simulink model "SISTEMA5_3"  (R2025b)
settings: Solver=VariableStepAuto  StartTime=0.0  StopTime=10.0  RelTol=1e-3
libraries: slpidlib x2

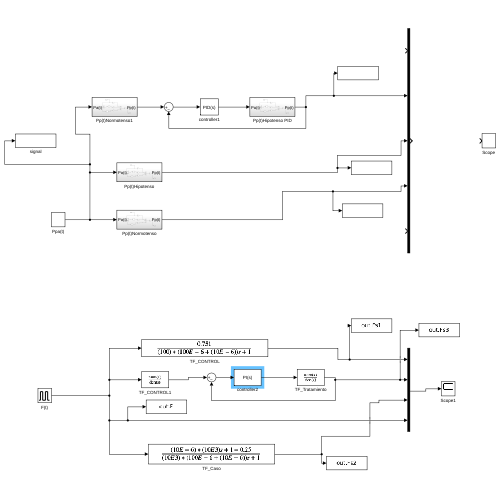
[thumbnail: Simulink's stored preview of the top-level diagram]
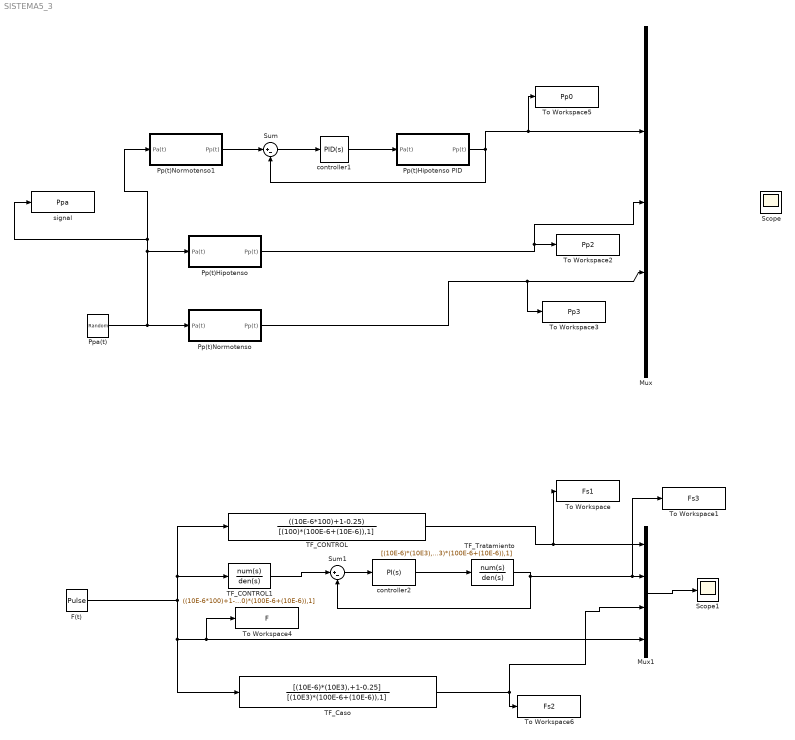
== system SISTEMA5_3 ==
  F(t) : DiscretePulseGenerator  PulseType=Time based  Period=10  PulseWidth=10  PhaseDelay=1
  Mux : Mux  Inputs=5
  Mux1 : Mux
  Pp(t)Hipotenso : Subsystem
  Pp(t)Hipotenso PID : Subsystem
  Pp(t)Normotenso : Subsystem
  Pp(t)Normotenso1 : Subsystem
  Ppa(t) : UniformRandomNumber  Minimum=-0.2  Seed=106  SampleTime=0.5
  Scope : Scope
  Scope1 : Scope
      settings: ActiveDisplayYMinimum=-0.12525889931530931  ActiveDisplayYMaximum=1.2530462249099128
  Sum : Sum  Inputs=|+-
  Sum1 : Sum  Inputs=|+-
  TF_CONTROL : TransferFcn  Numerator=((10E-6*100)+1-0.25)  Denominator=[(100)*(100E-6+(10E-6)),1]
  TF_CONTROL1 : TransferFcn  Numerator=((10E-6*100)+1-0.25)  Denominator=[(100)*(100E-6+(10E-6)),1]
  TF_Caso : TransferFcn  Numerator=[(10E-6)*(10E3),+1-0.25]  Denominator=[(10E3)*(100E-6+(10E-6)),1]
  TF_Tratamiento : TransferFcn  Numerator=[(10E-6)*(10E3),+1-0.25]  Denominator=[(10E3)*(100E-6+(10E-6)),1]
  To Workspace : ToWorkspace  VariableName=Fs1  SampleTime=-1
      settings: Save2DSignal=2-D array (concatenate along first dimension)
  To Workspace1 : ToWorkspace  VariableName=Fs3  SampleTime=-1
      settings: Save2DSignal=2-D array (concatenate along first dimension)
  To Workspace2 : ToWorkspace  VariableName=Pp2  SampleTime=-1
  To Workspace3 : ToWorkspace  VariableName=Pp3  SampleTime=-1
  To Workspace4 : ToWorkspace  VariableName=F  SampleTime=-1
      settings: Save2DSignal=2-D array (concatenate along first dimension)
  To Workspace5 : ToWorkspace  VariableName=Pp0  SampleTime=-1
  To Workspace6 : ToWorkspace  VariableName=Fs2  SampleTime=-1
      settings: Save2DSignal=2-D array (concatenate along first dimension)
  controller1 : slpidlib/PID Controller  Controller=PID  Form=Parallel  TimeDomain=Continuous-time  UseExternalTs=off  SampleTime=-1  IntegratorMethod=Forward Euler  FilterMethod=Forward Euler  ControllerParametersSource=internal  P=4.1264e-05  I=3267  UseKiTs=off  D=0  UseExternalDerivativeSource=off  N=100  UseFilter=on  TunerSelectOption=Transfer Function Based (PID Tuner App)  InitialConditionSource=internal  InitialConditionForIntegrator=0  InitialConditionForFilter=0  DifferentiatorICPrevScaledInput=0  ExternalReset=none  TrackingMode=off  Kt=1  LimitOutput=off  SatLimitsSource=internal  UpperSaturationLimit=inf  LowerSaturationLimit=-inf  LinearizeAsGain=on  AntiWindupMode=none  Kb=1  LimitIntegrator=off  UpperIntegratorSaturationLimit=inf  LowerIntegratorSaturationLimit=-inf  POutMin=[]  POutMax=[]  IOutMin=[]  IOutMax=[]  DOutMin=[]  DOutMax=[]  NOutMin=[]  NOutMax=[]  SumOutMin=[]  SumOutMax=[]  SaturationOutMin=[]  SaturationOutMax=[]  PParamMin=[]  PParamMax=[]  IParamMin=[]  IParamMax=[]  DParamMin=[]  DParamMax=[]  NParamMin=[]  NParamMax=[]  KbParamMin=[]  KbParamMax=[]  KtParamMin=[]  KtParamMax=[]  KbOutMin=[]  KbOutMax=[]  KtOutMin=[]  KtOutMax=[]  IntegratorOutMin=[]  IntegratorOutMax=[]  FilterOutMin=[]  FilterOutMax=[]  SumI1OutMin=[]  SumI1OutMax=[]  SumI2OutMin=[]  SumI2OutMax=[]  SumI3OutMin=[]  SumI3OutMax=[]  SumI4OutMin=[]  SumI4OutMax=[]  SumDOutMin=[]  SumDOutMax=[]  DifferentiatorOutMin=[]  DifferentiatorOutMax=[]  FilterDiffOutCoefMin=[]  FilterDiffOutCoefMax=[]  ReciprocalOutMin=[]  ReciprocalOutMax=[]  SumDenOutMin=[]  SumDenOutMax=[]  SumNumOutMin=[]  SumNumOutMax=[]  DivideOutMin=[]  DivideOutMax=[]  UdiffTsProdOutMin=[]  UdiffTsProdOutMax=[]  NTsProdOutMin=[]  NTsProdOutMax=[]  UintegralTsProdOutMin=[]  UintegralTsProdOutMax=[]  UngainTsProdOutMin=[]  UngainTsProdOutMax=[]  ClampingZeroOutDataTypeStr=Inherit: Inherit via back propagation  ClampingZeroOutMin=[]  ClampingZeroOutMax=[]  FilterDenConstantOutDataTypeStr=Inherit: Inherit via back propagation  FilterDenConstantOutMin=[]  FilterDenConstantOutMax=[]  PCopyOutDataTypeStr=Inherit: Inherit via back propagation  PCopyOutMin=[]  PCopyOutMax=[]  NCopyOutDataTypeStr=Inherit: Inherit via back propagation  NCopyOutMin=[]  NCopyOutMax=[]  IntegratorContinuousStateAttributes=''  IntegratorStateMustResolveToSignalObject=off  IntegratorRTWStateStorageClass=Auto  FilterContinuousStateAttributes=''  FilterStateMustResolveToSignalObject=off  FilterRTWStateStorageClass=Auto  ParallelPVariant=InternalParameters  IdealPVariant=Disabled  IVariant=InternalParameters  DVariant=InternalParameters  IntegratorVariant=Continuous  SatVariant=Disabled  AWVariant=Passthrough  PCopyVariant=Disabled  TRVariant=Disabled  FdbkBlocksVariant=Forward  IdealPFdbkVariant=Disabled  SatFdbkVariant=Disabled  DerivativeFilterVariant=ContFilter  NVariant=InternalParameters  NCopyVariant=Disabled  FilterICVariant=InternalICsFilter  IntegratorICVariant=InternalICs  ExternalResetVariant=Disabled  TRSumVariant=Passthrough  SumFdbkVariant=Disabled  SumVariant=Sum_PID  TsampFilterVariant=InternalTs  TsampNgainVariant=Passthrough  TsampIntegralVariant=Disabled_SignalSpec  ExternalSaturationOutDataTypeStr=Inherit: Same as second input  DerivativeSourceVariant=ErrorSignal  PreIntVariant=InternalPreInt
  controller2 : slpidlib/PID Controller  Controller=PI  Form=Parallel  TimeDomain=Continuous-time  UseExternalTs=off  SampleTime=-1  IntegratorMethod=Forward Euler  FilterMethod=Forward Euler  ControllerParametersSource=internal  P=0.0727508175898247  I=171448.180832654  UseKiTs=off  D=0  UseExternalDerivativeSource=off  N=100  UseFilter=on  TunerSelectOption=Transfer Function Based (PID Tuner App)  InitialConditionSource=internal  InitialConditionForIntegrator=0  InitialConditionForFilter=0  DifferentiatorICPrevScaledInput=0  ExternalReset=none  TrackingMode=off  Kt=1  LimitOutput=off  SatLimitsSource=internal  UpperSaturationLimit=inf  LowerSaturationLimit=-inf  LinearizeAsGain=on  AntiWindupMode=none  Kb=1  LimitIntegrator=off  UpperIntegratorSaturationLimit=inf  LowerIntegratorSaturationLimit=-inf  POutMin=[]  POutMax=[]  IOutMin=[]  IOutMax=[]  DOutMin=[]  DOutMax=[]  NOutMin=[]  NOutMax=[]  SumOutMin=[]  SumOutMax=[]  SaturationOutMin=[]  SaturationOutMax=[]  PParamMin=[]  PParamMax=[]  IParamMin=[]  IParamMax=[]  DParamMin=[]  DParamMax=[]  NParamMin=[]  NParamMax=[]  KbParamMin=[]  KbParamMax=[]  KtParamMin=[]  KtParamMax=[]  KbOutMin=[]  KbOutMax=[]  KtOutMin=[]  KtOutMax=[]  IntegratorOutMin=[]  IntegratorOutMax=[]  FilterOutMin=[]  FilterOutMax=[]  SumI1OutMin=[]  SumI1OutMax=[]  SumI2OutMin=[]  SumI2OutMax=[]  SumI3OutMin=[]  SumI3OutMax=[]  SumI4OutMin=[]  SumI4OutMax=[]  SumDOutMin=[]  SumDOutMax=[]  DifferentiatorOutMin=[]  DifferentiatorOutMax=[]  FilterDiffOutCoefMin=[]  FilterDiffOutCoefMax=[]  ReciprocalOutMin=[]  ReciprocalOutMax=[]  SumDenOutMin=[]  SumDenOutMax=[]  SumNumOutMin=[]  SumNumOutMax=[]  DivideOutMin=[]  DivideOutMax=[]  UdiffTsProdOutMin=[]  UdiffTsProdOutMax=[]  NTsProdOutMin=[]  NTsProdOutMax=[]  UintegralTsProdOutMin=[]  UintegralTsProdOutMax=[]  UngainTsProdOutMin=[]  UngainTsProdOutMax=[]  ClampingZeroOutDataTypeStr=Inherit: Inherit via back propagation  ClampingZeroOutMin=[]  ClampingZeroOutMax=[]  FilterDenConstantOutDataTypeStr=Inherit: Inherit via back propagation  FilterDenConstantOutMin=[]  FilterDenConstantOutMax=[]  PCopyOutDataTypeStr=Inherit: Inherit via back propagation  PCopyOutMin=[]  PCopyOutMax=[]  NCopyOutDataTypeStr=Inherit: Inherit via back propagation  NCopyOutMin=[]  NCopyOutMax=[]  IntegratorContinuousStateAttributes=''  IntegratorStateMustResolveToSignalObject=off  IntegratorRTWStateStorageClass=Auto  FilterContinuousStateAttributes=''  FilterStateMustResolveToSignalObject=off  FilterRTWStateStorageClass=Auto  ParallelPVariant=InternalParameters  IdealPVariant=Disabled  IVariant=InternalParameters  DVariant=Disabled  IntegratorVariant=Continuous  SatVariant=Disabled  AWVariant=Passthrough  PCopyVariant=Disabled  TRVariant=Disabled  FdbkBlocksVariant=Forward  IdealPFdbkVariant=Disabled  SatFdbkVariant=Disabled  DerivativeFilterVariant=Disabled  NVariant=Disabled  NCopyVariant=Disabled_SignalSpec  FilterICVariant=Disabled  IntegratorICVariant=InternalICs  ExternalResetVariant=Disabled  TRSumVariant=Passthrough  SumFdbkVariant=Disabled  SumVariant=Sum_PI  TsampFilterVariant=InternalTs  TsampNgainVariant=Passthrough  TsampIntegralVariant=Disabled_SignalSpec  ExternalSaturationOutDataTypeStr=Inherit: Same as second input  DerivativeSourceVariant=Disabled  PreIntVariant=InternalPreInt
  signal : ToWorkspace  VariableName=Ppa  SampleTime=-1
  wires:
  Pp(t)Normotenso1/1(Pp(t)) -> Sum/1
  Pp(t)Hipotenso/1(Pp(t)) -> Mux/3, To Workspace2/1
  Pp(t)Normotenso/1(Pp(t)) -> To Workspace3/1, Mux/4
  Sum/1 -> controller1/1
  Ppa(t)/1 -> Pp(t)Normotenso1/1(Pa(t)), signal/1, Pp(t)Hipotenso/1(Pa(t)), Pp(t)Normotenso/1(Pa(t))
  controller1/1 -> Pp(t)Hipotenso PID/1(Pa(t))
  Pp(t)Hipotenso PID/1(Pp(t)) -> To Workspace5/1, Mux/2, Sum/2
  TF_CONTROL/1 -> To Workspace/1, Mux1/1
  Mux1/1 -> Scope1/1
  controller2/1 -> TF_Tratamiento/1
  TF_CONTROL1/1 -> Sum1/1
  Sum1/1 -> controller2/1
  TF_Caso/1 -> Mux1/3, To Workspace6/1
  F(t)/1 -> TF_CONTROL/1, TF_CONTROL1/1, TF_Caso/1, To Workspace4/1, Mux1/4
  TF_Tratamiento/1 -> Sum1/2, To Workspace1/1, Mux1/2

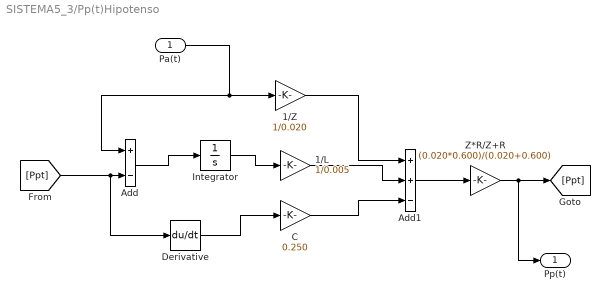
== system SISTEMA5_3/Pp(t)Hipotenso ==
  Pa(t) : Inport
  1/L : Gain  Gain=1/0.005
  1/Z : Gain  Gain=1/0.020
  Add : Sum  Inputs=+-
  Add1 : Sum  Inputs=++-
  C : Gain  Gain=0.250
  Derivative : Derivative
  Integrator : Integrator
  Z*R/Z+R : Gain  Gain=(0.020*0.600)/(0.020+0.600)
  Pp(t) : Outport
  wires:
  1/Z/1 -> Add1/1
  1/L/1 -> Add1/2
  C/1 -> Add1/3
  Add1/1 -> Z*R/Z+R/1
  Derivative/1 -> C/1
  Pa(t)/1 -> 1/Z/1, Add/1
  Z*R/Z+R/1 -> Pp(t)/1, [Ppt]
  [Ppt] -> Derivative/1, Add/2
  Add/1 -> Integrator/1
  Integrator/1 -> 1/L/1

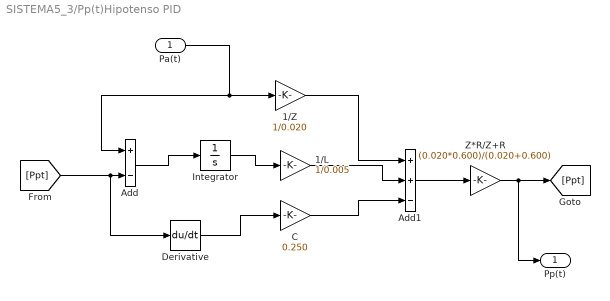
== system SISTEMA5_3/Pp(t)Hipotenso PID ==
  Pa(t) : Inport
  1/L : Gain  Gain=1/0.005
  1/Z : Gain  Gain=1/0.020
  Add : Sum  Inputs=+-
  Add1 : Sum  Inputs=++-
  C : Gain  Gain=0.250
  Derivative : Derivative
  Integrator : Integrator
  Z*R/Z+R : Gain  Gain=(0.020*0.600)/(0.020+0.600)
  Pp(t) : Outport
  wires:
  1/Z/1 -> Add1/1
  1/L/1 -> Add1/2
  C/1 -> Add1/3
  Add1/1 -> Z*R/Z+R/1
  Derivative/1 -> C/1
  Pa(t)/1 -> 1/Z/1, Add/1
  Z*R/Z+R/1 -> Pp(t)/1, [Ppt]
  [Ppt] -> Derivative/1, Add/2
  Add/1 -> Integrator/1
  Integrator/1 -> 1/L/1

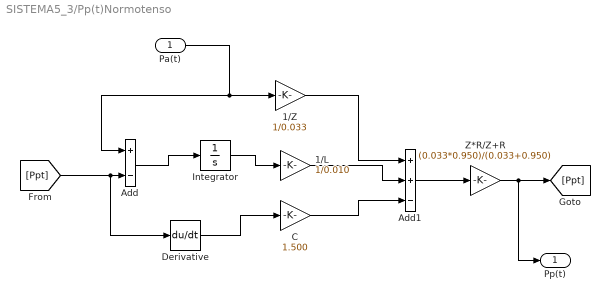
== system SISTEMA5_3/Pp(t)Normotenso ==
  Pa(t) : Inport
  1/L : Gain  Gain=1/0.010
  1/Z : Gain  Gain=1/0.033
  Add : Sum  Inputs=+-
  Add1 : Sum  Inputs=++-
  C : Gain  Gain=1.500
  Derivative : Derivative
  Integrator : Integrator
  Z*R/Z+R : Gain  Gain=(0.033*0.950)/(0.033+0.950)
  Pp(t) : Outport
  wires:
  1/Z/1 -> Add1/1
  1/L/1 -> Add1/2
  C/1 -> Add1/3
  Add1/1 -> Z*R/Z+R/1
  Derivative/1 -> C/1
  Pa(t)/1 -> 1/Z/1, Add/1
  Z*R/Z+R/1 -> Pp(t)/1, [Ppt]
  [Ppt] -> Derivative/1, Add/2
  Add/1 -> Integrator/1
  Integrator/1 -> 1/L/1

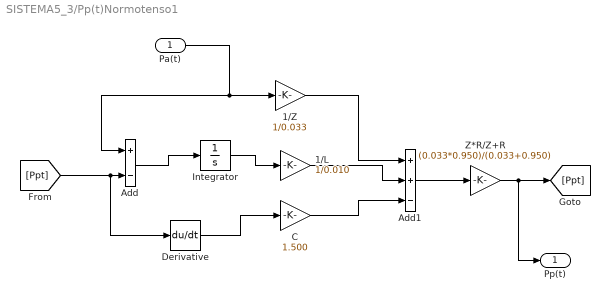
== system SISTEMA5_3/Pp(t)Normotenso1 ==
  Pa(t) : Inport
  1/L : Gain  Gain=1/0.010
  1/Z : Gain  Gain=1/0.033
  Add : Sum  Inputs=+-
  Add1 : Sum  Inputs=++-
  C : Gain  Gain=1.500
  Derivative : Derivative
  Integrator : Integrator
  Z*R/Z+R : Gain  Gain=(0.033*0.950)/(0.033+0.950)
  Pp(t) : Outport
  wires:
  1/Z/1 -> Add1/1
  1/L/1 -> Add1/2
  C/1 -> Add1/3
  Add1/1 -> Z*R/Z+R/1
  Derivative/1 -> C/1
  Pa(t)/1 -> 1/Z/1, Add/1
  Z*R/Z+R/1 -> Pp(t)/1, [Ppt]
  [Ppt] -> Derivative/1, Add/2
  Add/1 -> Integrator/1
  Integrator/1 -> 1/L/1
